simulink library "M5Core_Library"  (R2023a)
settings: Solver=VariableStepAuto  StartTime=0.0  StopTime=10.0  RelTol=1e-3
libraries: arduinolib x6
settings Model: Creator=auw_a  LastModifiedBy=auw_a

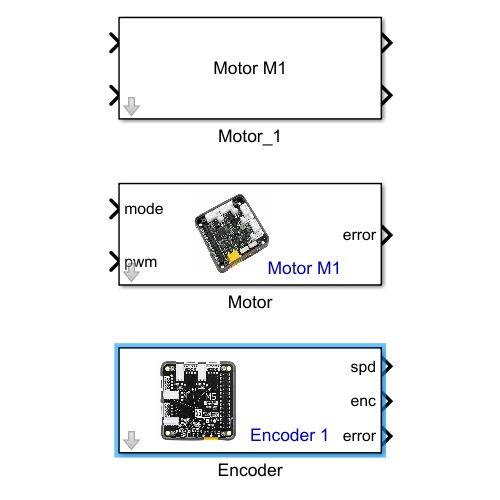
[thumbnail: Simulink's stored preview of the top-level diagram]
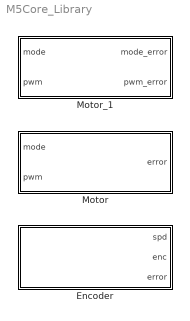
== system M5Core_Library ==
  Encoder : Subsystem  mask(Encoder - 4 Encoder DC Motor){M5_motor=1, s=0.01}
      mask prompts: M5_motor "Encoder channel:"; s "Sample Time:"
      mask help:
      | Measure the rotation of a motor in ticks.
      |
      | The block outputs the position and rotational speed of the motor. The position is measured in ticks and the speed is measured in ticks per 20ms of int32 data type.
      |
      | Every increment in the tick count indicates a clockwise rotation and every decrement in the tick count indicates a counterclockwise rotation.
      mask init:
      | switch M5_motor
      |     case '1'
      |         m = 0;
      |     case '2'
      |         m = 1;
      |     case '3'
      |         m = 2;
      |     case '4'
      |         m = 3;
      | end
      | str = "Encoder " + M5_motor;
      | label = str;
      mask Help:
      | PORTS
      | 
      | Output
      | 
      | Position - Position of rotating motor
      | scalar
      | The Position port outputs the relative change in the position of the rotating motor, measured in ticks.
      | Data Types: int32
      | 
      | Speed - Speed of rotating motor
      | scalar
      | The Speed port outputs the rotational speed of the motor, measured in ticks per 20 milli second.
      | Dependencies:
      | The Speed port is available only when you select the Show Speed output port parameter.
      | Data Types: int32
      | 
      | Output Port:
      | [2x1] array
      | Indicates that the block outputs the status of the I2C read operation at the output port. One for speed per 20ms and other for number of ticks.
      | The block outputs the status as a uint8 value. Each value corresponds to a data transfer status.
      | 
      | PARAMETERS
      | 
      | Encoder - Encoder channel number
      | 1 (default) | 2 | 3 | 4
      | Select the channel number of the encoder that is connected to the 4Encoder Motor Module.
      | 
      | Sample Time  - Time interval to read value fro encoder
      | 0.01 (default) |  -1 | non-negative real value
      | Specify how often the block reads the tick count from the encoder, in seconds. When you specify this parameter as -1, Simulink determines the best sample time for the block based on the block context within the model.
      mask TypeOptions M5_motor: 1 | 2 | 3 | 4
      mask Display:
      | im = imread('4EncoderModule.jpg');
      | image(im, [20, 5, 50, 50]);
      | color('blue');
      | text(75, 10, label);
  Motor : Subsystem  mask(Encoder DC Motor){M5_motor=M1}
      mask prompts: M5_motor "Motor Port:"
      mask help:
      | Set the speed and direction of the DC motor on the selected port.
      |
      | The block accepts an input between 127 to -127:
      | * 127 = Full speed forward
      | * 0 = Stop
      | * -127 = Full speed reverse
      mask init:
      | switch M5_motor
      |     case 'M1'
      |         m = 0;
      |     case 'M2'
      |         m = 1;
      |     case 'M3'
      |         m = 2;
      |     case 'M4'
      |         m = 3;
      | end
      | str = "Motor " + M5_motor;
      | label = str;
      mask Help:
      | The Motor DC Motors block controls the speed and direction of a DC motor connected to a MC4.0. The input signal determines the power supplied to the motor and the direction of rotation of the motor.
      | 
      | Supported Hardware
      | You can use the M1 M2 M3 M4 DC Motors block only with MC4.0 4Encoder Motor Module
      | 
      | PORTS
      | 
      | Input Port:
      | The sign of the input signal determines the direction of rotation of the DC motor. A positive sign indicates a forward rotation, whereas a negative sign indicates a reverse rotation. The amplitude determines the power supplied to the motor.
      | 
      | 1 to 127: Forward rotation, minimum to maximum power.
      | 
      | –1 to –127: Reverse rotation, minimum to maximum power.
      | 
      | 0: Stop.
      | 
      | Output Port:
      | [2x1] array
      | Indicates that the block outputs the status of the I2C write operation at the output port. One for mode and other for pwm.
      | The block outputs the status as a uint8 value. Each value corresponds to a data transfer status.
      | 
      | PARAMETERS
      | 
      | M5_motor - Port number on 4 Encoder Motor Module
      | M1 (default) | M2 | M3 | M4
      | Select the port number on the 4 Encoder Motor Module to which the DC motor is connected.
      mask TypeOptions M5_motor: M1 | M2 | M3 | M4
      mask Display:
      | im = imread('4EncoderMotorModule.jpg');
      | image(im, [40, 5, 50, 50]);
      | color('blue');
      | text(85, 10, label);
  Motor_1 : Subsystem  mask{M5_motor=M1}
      mask prompts: M5_motor "Motor Port"
      mask init:
      | switch M5_motor
      |     case 'M1'
      |         m = 0;
      |     case 'M2'
      |         m = 1;
      |     case 'M3'
      |         m = 2;
      |     case 'M4'
      |         m = 3;
      | end
      | str = "Motor " + M5_motor;
      | label = str;
      mask TypeOptions M5_motor: M1 | M2 | M3 | M4
      mask Display: disp(label);

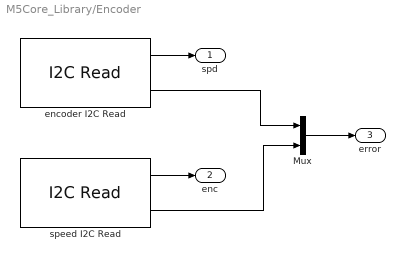
== system M5Core_Library/Encoder ==
  Mux : Mux  Inputs=2
  encoder I2C Read : arduinolib/I2C Read  I2CModule=0  Mode=Master  SlaveAddress=uint8(hex2dec('24'))  SlaveByteOrder=BigEndian  Direction=Receiver  RegisterAddressMode=on  RegisterAddress=uint8(hex2dec('40')) + m  SlaveDataType=int8  DataLength=1  NoAck=off  RepeatedStart=off  OutputStatus=on  blockPlatform=ARDUINO  SampleTime=s
  speed I2C Read : arduinolib/I2C Read  I2CModule=0  Mode=Master  SlaveAddress=uint8(hex2dec('24'))  SlaveByteOrder=BigEndian  Direction=Receiver  RegisterAddressMode=on  RegisterAddress=uint8(hex2dec('30')) + 4*m  SlaveDataType=int32  DataLength=1  NoAck=off  RepeatedStart=off  OutputStatus=on  blockPlatform=ARDUINO  SampleTime=s
  spd : Outport
  enc : Outport  Port=2
  error : Outport  Port=3
  wires:
  Mux/1 -> error/1
  speed I2C Read/2 -> Mux/2
  encoder I2C Read/2 -> Mux/1
  speed I2C Read/1 -> enc/1
  encoder I2C Read/1 -> spd/1

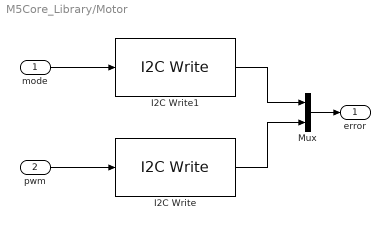
== system M5Core_Library/Motor ==
  mode : Inport
  pwm : Inport  Port=2
  I2C Write : arduinolib/I2C Write  I2CModule=0  Mode=Master  SlaveAddress=uint8(hex2dec('24'))  SlaveByteOrder=BigEndian  Direction=Transmitter  RegisterAddressMode=on  RegisterAddress=uint8(hex2dec('20')) + m  SlaveDataType=uint8  DataLength=1  NoAck=off  RepeatedStart=off  OutputStatus=on  blockPlatform=ARDUINO
  I2C Write1 : arduinolib/I2C Write  I2CModule=0  Mode=Master  SlaveAddress=uint8(hex2dec('24'))  SlaveByteOrder=BigEndian  Direction=Transmitter  RegisterAddressMode=on  RegisterAddress=uint8(hex2dec('60')) + m  SlaveDataType=uint8  DataLength=1  NoAck=off  RepeatedStart=off  OutputStatus=on  blockPlatform=ARDUINO
  Mux : Mux  Inputs=2
  error : Outport
  wires:
  Mux/1 -> error/1
  I2C Write/1 -> Mux/2
  I2C Write1/1 -> Mux/1
  pwm/1 -> I2C Write/1
  mode/1 -> I2C Write1/1

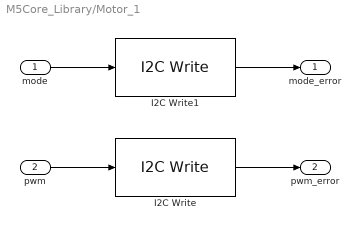
== system M5Core_Library/Motor_1 ==
  mode : Inport
  pwm : Inport  Port=2
  I2C Write : arduinolib/I2C Write  I2CModule=0  Mode=Master  SlaveAddress=uint8(hex2dec('24'))  SlaveByteOrder=BigEndian  Direction=Transmitter  RegisterAddressMode=on  RegisterAddress=uint8(hex2dec('20')) + m  SlaveDataType=uint8  DataLength=1  NoAck=off  RepeatedStart=off  OutputStatus=on  blockPlatform=ARDUINO
  I2C Write1 : arduinolib/I2C Write  I2CModule=0  Mode=Master  SlaveAddress=uint8(hex2dec('24'))  SlaveByteOrder=BigEndian  Direction=Transmitter  RegisterAddressMode=on  RegisterAddress=uint8(hex2dec('60')) + m  SlaveDataType=uint8  DataLength=1  NoAck=off  RepeatedStart=off  OutputStatus=on  blockPlatform=ARDUINO
  mode_error : Outport
  pwm_error : Outport  Port=2
  wires:
  I2C Write/1 -> pwm_error/1
  I2C Write1/1 -> mode_error/1
  pwm/1 -> I2C Write/1
  mode/1 -> I2C Write1/1
